simulink model "engine"  (R2020b)
settings: Solver=VariableStepAuto  StartTime=0.0  StopTime=10.0  RelTol=1e-3
undefined symbols (not defined in the file or in its folder): sigbuilder_block
settings Model: Creator=LaoZhu  LastModifiedBy=LaoZhu

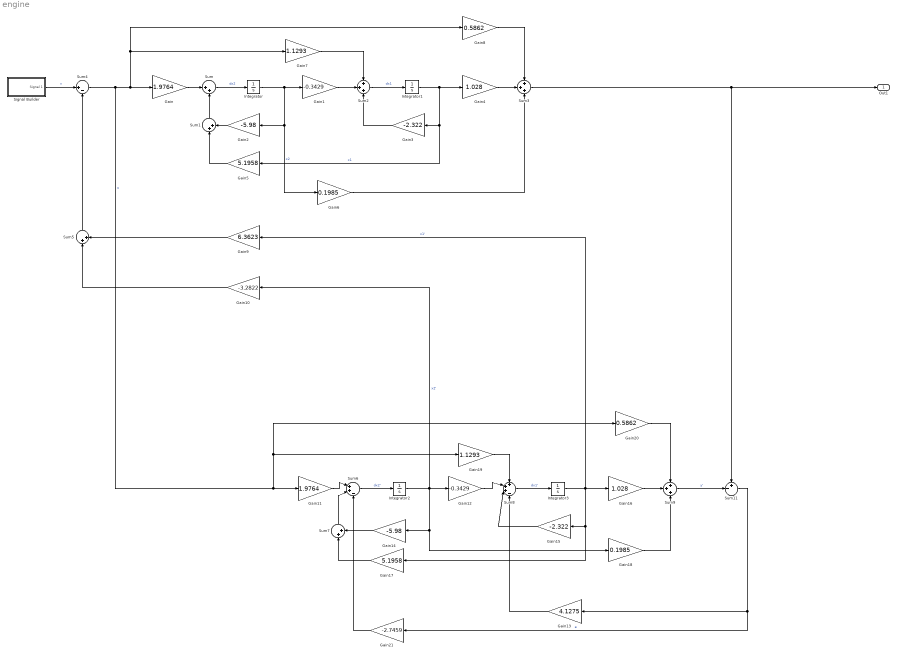
== system engine ==
  Gain : Gain  Gain=1.9764
  Gain1 : Gain  Gain=-0.3429
  Gain10 : Gain  Gain=-3.2822
  Gain11 : Gain  Gain=1.9764
  Gain12 : Gain  Gain=-0.3429
  Gain13 : Gain  Gain=4.1275
  Gain14 : Gain  Gain=-5.98
  Gain15 : Gain  Gain=-2.322
  Gain16 : Gain  Gain=1.028
  Gain17 : Gain  Gain=5.1958
  Gain18 : Gain  Gain=0.1985
  Gain19 : Gain  Gain=1.1293
  Gain2 : Gain  Gain=-5.98
  Gain20 : Gain  Gain=0.5862
  Gain21 : Gain  Gain=-2.7459
  Gain3 : Gain  Gain=-2.322
  Gain4 : Gain  Gain=1.028
  Gain5 : Gain  Gain=5.1958
  Gain6 : Gain  Gain=0.1985
  Gain7 : Gain  Gain=1.1293
  Gain8 : Gain  Gain=0.5862
  Gain9 : Gain  Gain=6.3623
  Integrator{,1..3} (4 alike) : Integrator
  Signal Builder : Subsystem  Tag=STV Subsys  LoadFcn=sigbuilder_block('load');  StartFcn=sigbuilder_block('start');  StopFcn=sigbuilder_block('stop');  ClipboardFcn=sigbuilder_block('clipboard');  mask(Sigbuilder block){tuvar=[0:10]}
      mask help: Simulink:masks:SigbuilderBlock_MD
      mask init:
      | if ~strcmp(get_param(bdroot(gcbh),'SimulationStatus'),'stopped') tuvar = sigbuilder_block('maskInit'); end
      settings: CopyFcn=sigbuilder_block('copy');  DeleteFcn=sigbuilder_block('delete');  ModelCloseFcn=sigbuilder_block('modelClose');  PreSaveFcn=sigbuilder_block('preSave');  PauseFcn=sigbuilder_block('pause');  ContinueFcn=sigbuilder_block('continue');  NameChangeFcn=sigbuilder_block('namechange');  OpenFcn=sigbuilder_block('open',[330 153.75 550.5 399.75 ]);  CloseFcn=sigbuilder_block('close');
      mask Display: plot(0, 0, 100, 100,[2, 2, 32, 32, 2], [68, 8, 8, 68, 68],[32, 2], [38, 38], [32, 19, 2],[53, 60, 44], [32, 17, 17, 2],[16, 16, 31, 31]);txt = getActiveGroup(gcbh);text(2, 100, txt,'verticalAlignment', 'top');
  Sum{,1,5,7} (4 alike) : Sum  Inputs=|++
  Sum11 : Sum  Inputs=+-|
  Sum2 : Sum  Inputs=+++
  Sum3 : Sum  Inputs=+++
  Sum4 : Sum  Inputs=|+-
  Sum6 : Sum  Inputs=|++-
  Sum8 : Sum  Inputs=+++-
  Sum9 : Sum  Inputs=+++
  Out1 : Outport  SignalName=y
  wires:
  Gain/1 -> Sum/1
  Sum/1 -> Integrator/1  "dx2"
  Integrator/1 -> Gain6/1, Gain2/1, Gain1/1  "x2"
  Gain2/1 -> Sum1/2
  Sum1/1 -> Sum/2
  Gain1/1 -> Sum2/2
  Sum2/1 -> Integrator1/1  "dx1"
  Integrator1/1 -> Gain4/1, Gain5/1, Gain3/1  "x1"
  Gain3/1 -> Sum2/3
  Gain4/1 -> Sum3/2
  Gain5/1 -> Sum1/1
  Gain6/1 -> Sum3/3
  Gain7/1 -> Sum2/1
  Gain8/1 -> Sum3/1
  Sum3/1 -> Sum11/1, Out1/1
  Sum4/1 -> Gain20/1, Gain19/1, Gain11/1, Gain8/1, Gain7/1, Gain/1  "u"
  Gain9/1 -> Sum5/2
  Gain10/1 -> Sum5/1
  Sum5/1 -> Sum4/2
  Gain17/1 -> Sum7/1
  Gain18/1 -> Sum9/3
  Sum8/1 -> Integrator3/1  "dx1'"
  Sum9/1 -> Sum11/2  "y'"
  Gain15/1 -> Sum8/3
  Gain19/1 -> Sum8/1
  Gain16/1 -> Sum9/2
  Gain14/1 -> Sum7/2
  Gain20/1 -> Sum9/1
  Gain11/1 -> Sum6/1
  Signal Builder/1(Signal 1) -> Sum4/1  "v"
  Sum7/1 -> Sum6/2
  Integrator3/1 -> Gain9/1, Gain16/1, Gain17/1, Gain15/1  "x1'"
  Sum6/1 -> Integrator2/1  "dx2'"
  Gain12/1 -> Sum8/2
  Integrator2/1 -> Gain10/1, Gain18/1, Gain14/1, Gain12/1  "x2'"
  Sum11/1 -> Gain21/1, Gain13/1  "e"
  Gain13/1 -> Sum8/4
  Gain21/1 -> Sum6/3

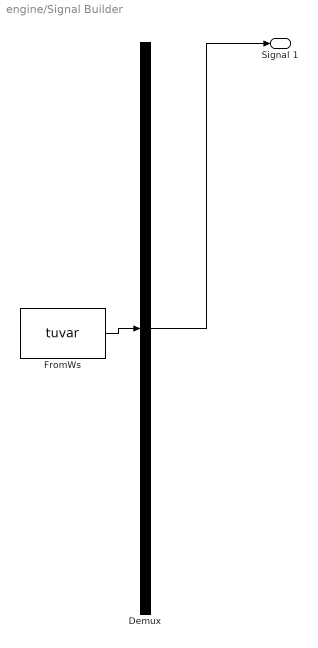
== system engine/Signal Builder ==
  Demux : Demux  Tag=STV Demux  Outputs=1
      settings: DisplayOption=none
  FromWs : FromWorkspace  Tag=STV FromWs  VariableName=tuvar
      SigBuilderData=|
      | common.afterFinalStr = 'Extrapolate'
      | common.sampleTime = 0
      | dataSet.timeRange = [0 10]
      | dataSet.name = 'Group 1'
      | sbobj.Groups.Name = 'Group 1'
      | sbobj.Groups.Signals.Name = 'Signal 1'
      | sbobj.Groups.Signals.XData = [0 0.05 1 3 3 5 5 7 7 10]
      | sbobj.Groups.Signals.YData = [0 0 0.1 0.1 0.2 0.2 0.3 0.3 0.5 0.5]
  Signal 1 : Outport  Tag=STV Outport
  wires:
  FromWs/1 -> Demux/1
  Demux/1 -> Signal 1/1
